simulink model "quadrocopter"  (Simulink 7.4)
settings: Solver=FixedStepDiscrete  StartTime=0.0  StopTime=30  FixedStep=0.001  RelTol=1e-3
values from neighbouring files (symbols this model uses):
  f1 = (I_y-I_z)/I_x    [quadrocopter_param.m]
  f2 = rot.J_z/I_x    [quadrocopter_param.m]
  f3 = (I_z-I_x)/I_y    [quadrocopter_param.m]
  f4 = rot.J_z/I_y    [quadrocopter_param.m]
  g = 9.81    [quadrocopter_param.m]
  I_x = elec.I_x+bat.I_x+2*boom.I_1x+2*boom.I_1y+2*mot.I_1x+2*mot.I_1y+                             2*rot.I_1x+2*rot.I_1y    [quadrocopter_param.m]
  I_y = elec.I_y+bat.I_y+2*boom.I_1x+2*boom.I_1y+2*mot.I_1x+2*mot.I_1y+                             2*rot.I_1x+2*rot.I_1y    [quadrocopter_param.m]
  I_z = elec.I_z+bat.I_z+4*boom.I_1z+4*mot.I_1x+4*rot.I_1x    [quadrocopter_param.m]
  m = elec.m+bat.m+boom.m+mot.m+rot.m    [quadrocopter_param.m]
  speed = rpm.*2*pi/60    [quadrocopter_param.m]
  thrust = [0.58 1 1.33 2 2.54 3.33 4.08 4.54]    [quadrocopter_param.m]
  Ts = 0.001    [quadrocopter_param.m]
undefined symbols (not defined in the file or in its folder): boom, DiscIntNeverNeededParam
libraries: simulink x2, dspinverses x1
settings Model: Creator=Joachim  LastModifiedBy=Joachim
settings DataIOCC: LimitDataPoints=off  MaxDataPoints=10000  SaveFinalState=on  SaveState=on

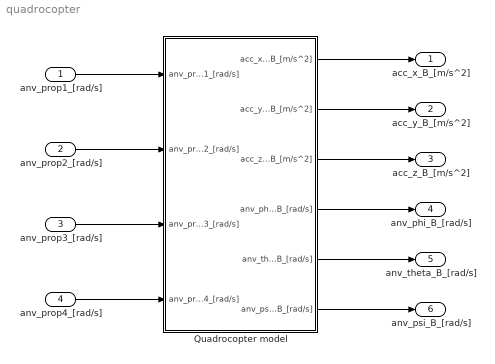
== system quadrocopter ==
  anv_prop1_[rad/s] : Inport  OutDataType=fixdt(1, 16)  OutScaling=2^0
  anv_prop2_[rad/s] : Inport  Port=2  OutDataType=fixdt(1, 16)  OutScaling=2^0
  anv_prop3_[rad/s] : Inport  Port=3  OutDataType=fixdt(1, 16)  OutScaling=2^0
  anv_prop4_[rad/s] : Inport  Port=4  OutDataType=fixdt(1, 16)  OutScaling=2^0
  Quadrocopter model : Subsystem
  acc_x_B_[m/s^2] : Outport  OutDataType=fixdt(1, 16)  OutScaling=2^0
  acc_y_B_[m/s^2] : Outport  Port=2  OutDataType=fixdt(1, 16)  OutScaling=2^0
  acc_z_B_[m/s^2] : Outport  Port=3  OutDataType=fixdt(1, 16)  OutScaling=2^0
  anv_phi_B_[rad/s] : Outport  Port=4  OutDataType=fixdt(1, 16)  OutScaling=2^0
  anv_theta_B_[rad/s] : Outport  Port=5  OutDataType=fixdt(1, 16)  OutScaling=2^0
  anv_psi_B_[rad/s] : Outport  Port=6  OutDataType=fixdt(1, 16)  OutScaling=2^0
  wires:
  Quadrocopter model/1(acc_x_B_[m/s^2]) -> acc_x_B_[m/s^2]/1
  Quadrocopter model/2(acc_y_B_[m/s^2]) -> acc_y_B_[m/s^2]/1
  Quadrocopter model/3(acc_z_B_[m/s^2]) -> acc_z_B_[m/s^2]/1
  Quadrocopter model/4(anv_phi_B_[rad/s]) -> anv_phi_B_[rad/s]/1
  Quadrocopter model/5(anv_theta_B_[rad/s]) -> anv_theta_B_[rad/s]/1
  Quadrocopter model/6(anv_psi_B_[rad/s]) -> anv_psi_B_[rad/s]/1
  anv_prop1_[rad/s]/1 -> Quadrocopter model/1(anv_prop1_[rad/s])
  anv_prop2_[rad/s]/1 -> Quadrocopter model/2(anv_prop2_[rad/s])
  anv_prop3_[rad/s]/1 -> Quadrocopter model/3(anv_prop3_[rad/s])
  anv_prop4_[rad/s]/1 -> Quadrocopter model/4(anv_prop4_[rad/s])

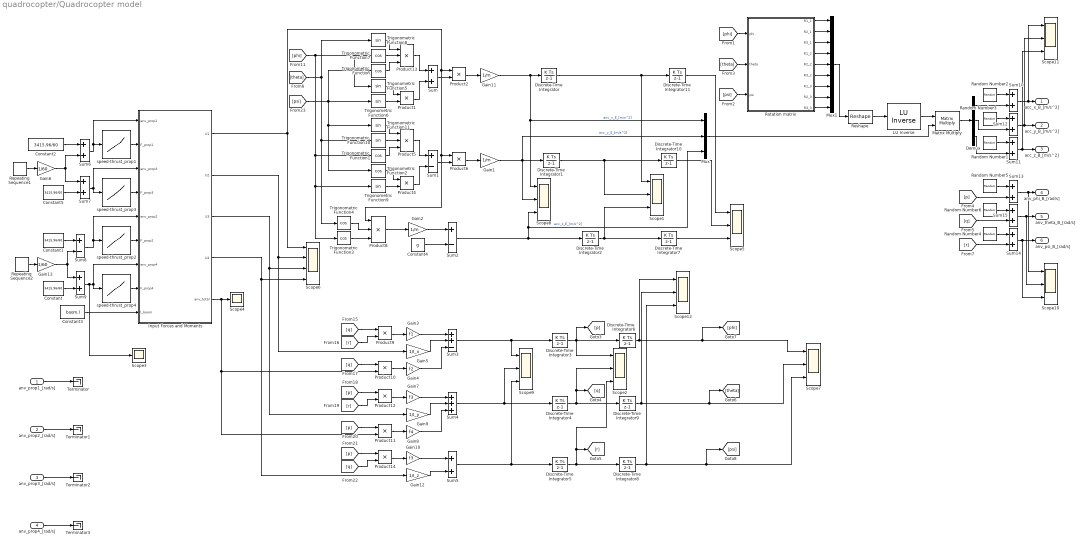
== system quadrocopter/Quadrocopter model ==
  anv_prop1_[rad/s] : Inport  OutDataType=fixdt(1, 16)  OutScaling=2^0
  anv_prop2_[rad/s] : Inport  Port=2  OutDataType=fixdt(1, 16)  OutScaling=2^0
  anv_prop3_[rad/s] : Inport  Port=3  OutDataType=fixdt(1, 16)  OutScaling=2^0
  anv_prop4_[rad/s] : Inport  Port=4  OutDataType=fixdt(1, 16)  OutScaling=2^0
  " LU Inverse" : dspinverses/ LU Inverse  SystemSampleTime=-1
  Constant{,1..2,5} (4 alike) : Constant  Value=3415.96/60  OutDataType=fixdt(1, 16)  OutScaling=2^0
  Constant3 : Constant  Value=boom.l  OutDataType=fixdt(1, 16)  OutScaling=2^0
  Constant4 : Constant  Value=g  OutDataType=fixdt(1, 16)  OutScaling=2^0
  Demux : Demux  Outputs=3
  Discrete-Time Integrator{,1..11} (12 alike) : DiscreteIntegrator  SampleTime=Ts  OutDataType=fixdt(1, 16)  OutScaling=2^0  ICPrevOutput=DiscIntNeverNeededParam  ICPrevScaledInput=DiscIntNeverNeededParam
  Gain1 : Gain  Gain=1/m  ParameterDataType=fixdt(1, 16)  ParameterScaling=2^0  OutDataType=fixdt(1, 16)  OutScaling=2^0
  Gain10 : Gain  Gain=f3  ParameterDataType=fixdt(1, 16)  ParameterScaling=2^0  OutDataType=fixdt(1, 16)  OutScaling=2^0
  Gain11 : Gain  Gain=1/m  ParameterDataType=fixdt(1, 16)  ParameterScaling=2^0  OutDataType=fixdt(1, 16)  OutScaling=2^0
  Gain12 : Gain  Gain=1/I_z  ParameterDataType=fixdt(1, 16)  ParameterScaling=2^0  OutDataType=fixdt(1, 16)  OutScaling=2^0
  Gain13 : Gain  Gain=1/60  ParameterDataType=fixdt(1, 16)  ParameterScaling=2^0  OutDataType=fixdt(1, 16)  OutScaling=2^0
  Gain2 : Gain  Gain=1/m  ParameterDataType=fixdt(1, 16)  ParameterScaling=2^0  OutDataType=fixdt(1, 16)  OutScaling=2^0
  Gain3 : Gain  Gain=f1  ParameterDataType=fixdt(1, 16)  ParameterScaling=2^0  OutDataType=fixdt(1, 16)  OutScaling=2^0
  Gain4 : Gain  Gain=f2  ParameterDataType=fixdt(1, 16)  ParameterScaling=2^0  OutDataType=fixdt(1, 16)  OutScaling=2^0
  Gain5 : Gain  Gain=1/I_x  ParameterDataType=fixdt(1, 16)  ParameterScaling=2^0  OutDataType=fixdt(1, 16)  OutScaling=2^0
  Gain6 : Gain  Gain=1/60  ParameterDataType=fixdt(1, 16)  ParameterScaling=2^0  OutDataType=fixdt(1, 16)  OutScaling=2^0
  Gain7 : Gain  Gain=f3  ParameterDataType=fixdt(1, 16)  ParameterScaling=2^0  OutDataType=fixdt(1, 16)  OutScaling=2^0
  Gain8 : Gain  Gain=f4  ParameterDataType=fixdt(1, 16)  ParameterScaling=2^0  OutDataType=fixdt(1, 16)  OutScaling=2^0
  Gain9 : Gain  Gain=1/I_y  ParameterDataType=fixdt(1, 16)  ParameterScaling=2^0  OutDataType=fixdt(1, 16)  OutScaling=2^0
  Input Forces and Moments : Stateflow chart
  Matrix Multiply : Product  Multiplication=Matrix(*)  OutDataType=sfix(16)  OutScaling=2^0
  Mux : Mux  Inputs=3
  Mux1 : Mux  Inputs=9
  Product{1..2,4,6,9..12,14} (9 alike) : Product  OutDataType=fixdt(1, 16)  OutScaling=2^0  RndMeth=Zero
  Product13 : Product  Inputs=3  OutDataType=fixdt(1, 16)  OutScaling=2^0  RndMeth=Zero
  Product5 : Product  Inputs=3  OutDataType=fixdt(1, 16)  OutScaling=2^0  RndMeth=Zero
  Product8 : Product  Inputs=3  OutDataType=fixdt(1, 16)  OutScaling=2^0  RndMeth=Zero
  Random Number{1..6} (6 alike) : RandomNumber  Variance=0.05  SampleTime=Ts
  Repeating Sequence1 : simulink/Sources/Repeating Sequence  SystemSampleTime=-1  rep_seq_t=[0 1 2 5 6 7 8 9 10 30]  rep_seq_y="[0 0 0  0 0 0 0 0 0 0]"
  Repeating Sequence2 : simulink/Sources/Repeating Sequence  SystemSampleTime=-1  rep_seq_t=[0 1 2 5 6 7 8 9 10 30]  rep_seq_y="[0 10 0  0 -10 0 0 0 0 0]"
  Reshape : Reshape  OutputDimensionality=Customize  OutputDimensions=[3,3]
  Rotation matrix : Stateflow chart
  Scope{1..2,5,7..12} (9 alike) : Scope  NumInputPorts=3
      Scope1 settings: YMin=-5~-5~-5  YMax=5~5~5
      Scope10 settings: YMin=-5~-5~-5  YMax=5~5~5  SaveName=ScopeData9
      Scope11 settings: YMin=-5~-5~-5  YMax=5~5~5  SaveName=ScopeData10
      Scope12 settings: YMin=-5~-5~-5  YMax=5~5~5  SaveName=ScopeData11
      Scope2 settings: YMin=-5~-5~-5  YMax=5~5~5
      Scope5 settings: YMin=-5~-5~-5  YMax=5~5~5  SaveName=ScopeData3
      Scope7 settings: YMin=-5~-5~-5  YMax=5~5~5  SaveName=ScopeData6
      Scope8 settings: TimeRange=20  YMin=-1.8~0~-12  YMax=0.2~10~2  SaveName=ScopeData7
      Scope9 settings: YMin=-5~-5~-5  YMax=5~5~5  SaveName=ScopeData8
  Scope3 : Scope
      settings: TimeRange=10  YMin=100  YMax=200  SaveName=ScopeData2
  Scope4 : Scope
      settings: SaveName=ScopeData4
  Scope6 : Scope  NumInputPorts=4
      settings: YMin=-5~-5~-5~-5  YMax=5~5~5~5  SaveName=ScopeData5
  Sum{,5..7,9..15} (11 alike) : Sum  OutDataType=fixdt(1, 16)  OutScaling=2^0
  Sum1 : Sum  Inputs=+-  OutDataType=fixdt(1, 16)  OutScaling=2^0
  Sum2 : Sum  Inputs=+-  OutDataType=fixdt(1, 16)  OutScaling=2^0
  Sum3 : Sum  Inputs=++-  OutDataType=fixdt(1, 16)  OutScaling=2^0
  Sum4 : Sum  Inputs=+++  OutDataType=fixdt(1, 16)  OutScaling=2^0
  Sum8 : Sum  Inputs=+-  OutDataType=fixdt(1, 16)  OutScaling=2^0
  Terminator{,1..3} (4 alike) : Terminator
  Trigonometric Function{,1..4,7} (6 alike) : Trigonometry  Operator=cos
  Trigonometric Function{5..6,8..11} (6 alike) : Trigonometry
  speed-thrust_prop{1..4} (4 alike) : Lookup  InputValues=speed  Table=thrust  OutDataType=fixdt(1, 16)  OutScaling=2^0
  acc_x_B_[m/s^2] : Outport  OutDataType=fixdt(1, 16)  OutScaling=2^0
  acc_y_B_[m/s^2] : Outport  Port=2  OutDataType=fixdt(1, 16)  OutScaling=2^0
  acc_z_B_[m/s^2] : Outport  Port=3  OutDataType=fixdt(1, 16)  OutScaling=2^0
  anv_phi_B_[rad/s] : Outport  Port=4  OutDataType=fixdt(1, 16)  OutScaling=2^0
  anv_theta_B_[rad/s] : Outport  Port=5  OutDataType=fixdt(1, 16)  OutScaling=2^0
  anv_psi_B_[rad/s] : Outport  Port=6  OutDataType=fixdt(1, 16)  OutScaling=2^0
  wires:
  speed-thrust_prop1/1 -> Input Forces and Moments/2(F_prop1)
  speed-thrust_prop4/1 -> Input Forces and Moments/8(F_prop4)
  Discrete-Time Integrator5/1 -> [r], Scope2/3, Discrete-Time Integrator8/1
  Discrete-Time Integrator4/1 -> [q], Scope2/2, Discrete-Time Integrator9/1
  Discrete-Time Integrator3/1 -> [p], Discrete-Time Integrator6/1, Scope2/1
  Discrete-Time Integrator8/1 -> Scope12/3, [psi], Scope7/3
  Discrete-Time Integrator9/1 -> Scope12/2, [theta], Scope7/2
  Discrete-Time Integrator6/1 -> Scope12/1, [phi], Scope7/1
  Input Forces and Moments/5(anv_total) -> Scope4/1, Product10/2, Product11/2
  [q] -> Product9/1
  [r] -> Product9/2
  Product9/1 -> Gain3/1
  Gain3/1 -> Sum3/1
  [q] -> Product10/1
  Product10/1 -> Gain4/1
  Input Forces and Moments/2(U2) -> Gain5/1, Scope6/2
  Gain5/1 -> Sum3/2
  Gain4/1 -> Sum3/3
  Sum3/1 -> Discrete-Time Integrator3/1, Scope9/1
  Input Forces and Moments/1(U1) -> Scope6/1, Product2/1, Product6/1, Product8/1
  [p] -> Product12/1
  [r] -> Product12/2
  Product12/1 -> Gain7/1
  Gain7/1 -> Sum4/1
  [p] -> Product11/1
  Product11/1 -> Gain8/1
  Gain9/1 -> Sum4/2
  Gain8/1 -> Sum4/3
  Input Forces and Moments/3(U3) -> Gain9/1, Scope6/3
  Sum4/1 -> Discrete-Time Integrator4/1, Scope9/2
  [p] -> Product14/1
  [q] -> Product14/2
  Product14/1 -> Gain10/1
  Gain10/1 -> Sum5/1
  Gain12/1 -> Sum5/2
  Input Forces and Moments/4(U4) -> Gain12/1, Scope6/4
  Sum5/1 -> Discrete-Time Integrator5/1, Scope9/3
  Constant3/1 -> Input Forces and Moments/9(l_boom)
  Discrete-Time Integrator7/1 -> Scope5/3
  Discrete-Time Integrator10/1 -> Scope5/2
  Discrete-Time Integrator11/1 -> Scope5/1
  Sum2/1 -> Discrete-Time Integrator2/1, Scope8/3, Mux/3  "acc_z_E_[m/s^2]"
  Product8/1 -> Gain2/1
  [phi] -> Trigonometric Function5/1, Trigonometric Function7/1, Trigonometric Function1/1, Trigonometric Function3/1, Trigonometric Function9/1
  Gain1/1 -> Discrete-Time Integrator1/1, Scope8/2, Mux/2  "acc_y_E_[m/s^2]"
  [theta] -> Trigonometric Function8/1, Trigonometric Function4/1, Trigonometric Function10/1
  Discrete-Time Integrator2/1 -> Scope1/3, Discrete-Time Integrator7/1
  Discrete-Time Integrator1/1 -> Scope1/2, Discrete-Time Integrator10/1
  Discrete-Time Integrator/1 -> Scope1/1, Discrete-Time Integrator11/1
  [psi] -> Trigonometric Function6/1, Trigonometric Function/1, Trigonometric Function11/1, Trigonometric Function2/1
  Trigonometric Function6/1 -> Product1/2
  Trigonometric Function5/1 -> Product1/1
  Product1/1 -> Sum/2
  Trigonometric Function8/1 -> Product13/1
  Trigonometric Function7/1 -> Product13/2
  Trigonometric Function/1 -> Product13/3
  Product13/1 -> Sum/1
  Sum/1 -> Product2/2
  Product2/1 -> Gain11/1
  Trigonometric Function9/1 -> Product4/2
  Trigonometric Function2/1 -> Product4/1
  Product4/1 -> Sum1/2
  Trigonometric Function11/1 -> Product5/1
  Trigonometric Function10/1 -> Product5/2
  Trigonometric Function1/1 -> Product5/3
  Product5/1 -> Sum1/1
  Sum1/1 -> Product6/2
  Product6/1 -> Gain1/1
  Gain11/1 -> Discrete-Time Integrator/1, Scope8/1, Mux/1  "acc_x_E_[m/s^2]"
  Gain2/1 -> Sum2/1
  Trigonometric Function3/1 -> Product8/3
  Trigonometric Function4/1 -> Product8/2
  Constant4/1 -> Sum2/2
  Constant2/1 -> Sum6/1
  Repeating Sequence1/1 -> Gain6/1
  Sum6/1 -> speed-thrust_prop1/1, Input Forces and Moments/1(anv_prop1)
  Constant5/1 -> Sum7/2
  Sum7/1 -> speed-thrust_prop3/1, Input Forces and Moments/3(anv_prop3)
  [phi] -> Rotation matrix/1(phi)
  [theta] -> Rotation matrix/2(theta)
  [psi] -> Rotation matrix/3(psi)
  Rotation matrix/1(R1_1) -> Mux1/1
  Rotation matrix/2(R2_1) -> Mux1/2
  Rotation matrix/3(R3_1) -> Mux1/3
  Rotation matrix/4(R1_2) -> Mux1/4
  Rotation matrix/5(R2_2) -> Mux1/5
  Rotation matrix/6(R3_2) -> Mux1/6
  Rotation matrix/7(R1_3) -> Mux1/7
  Rotation matrix/8(R2_3) -> Mux1/8
  Rotation matrix/9(R3_3) -> Mux1/9
  Mux1/1 -> Reshape/1
  Mux/1 -> Matrix Multiply/2
  Reshape/1 -> " LU Inverse"/1
  Repeating Sequence2/1 -> Gain13/1
  Constant1/1 -> Sum8/1
  Constant/1 -> Sum9/2
  Sum9/1 -> speed-thrust_prop4/1, Input Forces and Moments/7(anv_prop4), Scope3/1
  Sum8/1 -> speed-thrust_prop2/1, Input Forces and Moments/5(anv_prop2)
  Matrix Multiply/1 -> Demux/1
  Random Number2/1 -> Sum10/1
  Demux/1 -> Sum10/2
  Random Number1/1 -> Sum11/1
  Demux/3 -> Sum11/2
  Random Number3/1 -> Sum12/1
  Demux/2 -> Sum12/2
  Sum10/1 -> acc_x_B_[m/s^2]/1, Scope11/1
  Sum12/1 -> acc_y_B_[m/s^2]/1, Scope11/2
  Sum11/1 -> acc_z_B_[m/s^2]/1, Scope11/3
  Random Number5/1 -> Sum13/1
  [p] -> Sum13/2
  Random Number4/1 -> Sum14/1
  [r] -> Sum14/2
  Random Number6/1 -> Sum15/1
  [q] -> Sum15/2
  Sum13/1 -> anv_phi_B_[rad/s]/1, Scope10/1
  Sum15/1 -> anv_theta_B_[rad/s]/1, Scope10/2
  Sum14/1 -> anv_psi_B_[rad/s]/1, Scope10/3
  anv_prop4_[rad/s]/1 -> Terminator3/1
  anv_prop3_[rad/s]/1 -> Terminator2/1
  anv_prop2_[rad/s]/1 -> Terminator1/1
  anv_prop1_[rad/s]/1 -> Terminator/1
  Gain6/1 -> Sum6/2, Sum7/1
  Gain13/1 -> Sum9/1, Sum8/2
  speed-thrust_prop3/1 -> Input Forces and Moments/4(F_prop3)
  speed-thrust_prop2/1 -> Input Forces and Moments/6(F_prop2)
  " LU Inverse"/1 -> Matrix Multiply/1

== matlab function Quadrocopter model/Rotation matrix ==
  data: phi input double; theta input double; psi input double; R1_1 output double; R2_1 output double; R3_1 output double; R1_2 output double; R2_2 output double; R3_2 output double; R1_3 output double; R2_3 output double; R3_3 output double
function [ R1_1, R2_1, R3_1, R1_2, R2_2, R3_2, R1_3, R2_3, R3_3] = input...
                                                    (phi, theta, psi)
% Transformation of E-frame to B-Frame
R1_1 = cos(psi)*cos(theta);
R2_1 = sin(psi)*cos(theta);
R3_1 = -sin(theta);
R1_2 = -sin(psi)*cos(phi)+cos(psi)*sin(theta)*sin(phi);
R2_2 = cos(psi)*cos(phi)+sin(psi)*sin(theta)*sin(phi);
R3_2 = cos(theta)*sin(phi);
R1_3 = sin(psi)*sin(phi)+cos(psi)*sin(theta)*cos(phi);
R2_3 = -cos(psi)*sin(phi)+sin(psi)*sin(theta)*cos(phi);
R3_3 = cos(theta)*cos(phi);

== matlab function Quadrocopter model/Input Forces and Moments ==
  data: anv_prop1 input double; F_prop1 input double; anv_prop3 input double; F_prop3 input double; anv_prop2 input double; F_prop2 input double; anv_prop4 input double; U1 output double; F_prop4 input double; U2 output double; U3 output double; U4 output double; l_boom input double; anv_total output double
function [U1, U2, U3, U4, anv_total] = input(anv_prop1,F_prop1,anv_prop3,...
    F_prop3,anv_prop2,F_prop2,anv_prop4,F_prop4,l_boom)
%#eml

% Calculating Thrust in z-axis with respect to body fixed coordinate system
U1 = F_prop1 + F_prop2 + F_prop3 + F_prop4;             % [N]

% Calculating Torque around x-axis (Roll) due to Thrust
U2 = l_boom*(-F_prop4+F_prop2);                         % [Nm]

% Calculating Torque around y-axis (Pitch) due to Thrust
U3 = l_boom*(-F_prop1+F_prop3);                         % [Nm]

% Calculating Torque around z-axis (Yaw) due to Thrust
U4 = l_boom*(F_prop1-F_prop2+F_prop3-F_prop4);          % [Nm]

% Overall propeller speed
anv_total = anv_prop1-anv_prop2+anv_prop3-anv_prop4;    % [rad/s]
